simulink library "Vapour_Content"  (R2018b)
settings: Solver=ode45  StartTime=0.0  StopTime=10.0  RelTol=1e-3  EnableMultiTasking=on
undefined symbols (not defined in the file): CarnotCallbacks_Vapour_Content
settings Model: Creator=lena.frank  LastModifiedBy=P41573
settings DataIOCC: LimitDataPoints=on  SaveFormat=Array  SignalLoggingSaveFormat=ModelDataLogs
settings OptimizationCC: ExpressionDepthLimit=2147483647  LifeSpan=inf
settings DebuggingCC: UnderspecifiedInitializationDetection=Classic  MergeDetectMultiDrivingBlocksExec=none  SolverPrmCheckMsg=warning  FcnCallInpInsideContextMsg=warning  StateNameClashWarn=warning  SFUnexpectedBacktrackingDiag=warning  SFNoUnconditionalDefaultTransitionDiag=warning  SFExecutionAtInitializationDiag=none
settings HardwareCC: ProdBitPerPointer=32  ProdBitPerSizeT=32  ProdBitPerPtrDiffT=32  ProdLargestAtomicFloat=None  ProdIntDivRoundTo=Undefined  ProdEndianess=Unspecified  ProdWordSize=32  ProdHWDeviceType=32-bit Generic
settings ModelReferenceCC: PropagateSignalLabelsOutOfModel=off
settings SFSimCC: SimUseLocalCustomCode=off
settings RTWCC: RTWUseLocalCustomCode=off
settings CodeAppCC: StateflowObjectComments=on
settings GRTTargetCC: TargetLangStandard=C89/C90 (ANSI)  GeneratePreprocessorConditionals=Disable all  CombineOutputUpdateFcns=off  GRTInterface=on
settings ConfigComp: CovMetricSettings=dw  CovHtmlReporting=on  CovSaveCumulativeToWorkspaceVar=on  CovSaveSingleToWorkspaceVar=on  CovExternalEMLEnable=off

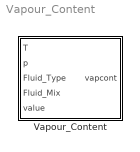
== system Vapour_Content ==
  Vapour_Content : Subsystem  LoadFcn=CarnotCallbacks_Vapour_Content('LoadFcn');  InitFcn=load('THB.mat');  VariantControl=CarlibClassic  mask(vapourcontent){INPUTARGUMENTS=state variables (classic), PROPERTYTYPE=density, DEBUGLEVEL=WARNINGLEVEL, MAXTOTALMESSAGES=inf, MAXCONSECUTIVEMESSAGES=inf, WRITETOFILE=0, FILENAME='errors.txt'}
      mask prompts: INPUTARGUMENTS "Input arguments"; PROPERTYTYPE "property type"; DEBUGLEVEL "Debug level"; MAXTOTALMESSAGES "maximum number of total warning"; MAXCONSECUTIVEMESSAGES "maximum number of consecutive warnings"; WRITETOFILE "write messages to file"; FILENAME "filename for error messages"
      mask help:
      | The block calculates the (water-)vapour content of water or water-glycol mixture by the value of a specified property. The block calls the function "vapourcontent" in the CARNOT library "Carlib".
      | Temperature and the "Value" may be a scalar or vector, all other inputs must be scalar (length of "temperature" and "value" must be same).
      | You may use the block "GlobalMessageLevel" in the Toolbox to handle the debugging messages.
      | Definition of property-types
      | property                    unit
      |  density                     [kg/m³]
      |  heat capacity           [J/kgK]
      |  heat conductivity     [W/mK]
      |  kinematic viscosity   [m²/s]
      |  enthalpy                   [J/kg]
      |  entropy                     [J/kgK]
      |  prandtl                      [-]
      |  specific volume        [m³/kg]
      mask init:
      | %Inports
      | CarnotCallbacks_Vapour_Content('CreateInports');
      | 
      | %global debug level
      | [DEBUGLEVEL, MAXTOTALMESSAGES, MAXCONSECUTIVEMESSAGES, WRITETOFILE, FILENAME] = CarnotCallbacks_Vapour_Content('CheckDebugLevels', DEBUGLEVEL, MAXTOTALMESSAGES, MAXCONSECUTIVEMESSAGES, WRITETOFILE, FILENAME);
      mask Help: web(fullfile(path_carnot('help'),'vapour_content.html'),'-helpbrowser')
      mask TypeOptions INPUTARGUMENTS: state variables (classic) | THB | THV
      mask Callback INPUTARGUMENTS: CarnotCallbacks_Vapour_Content('MaskVisibilities');
      mask TypeOptions PROPERTYTYPE: density | heat capacity | heat conductivity | kinematic viscosity | enthalpy | entropy | prandtl | specific volume
      mask TypeOptions DEBUGLEVEL: DEBUGLEVEL | INFOLEVEL | WARNINGLEVEL | ERRORLEVEL | FATALLEVEL | NOLEVEL
      mask DialogControl ParameterTabVar0 Prompt: Parameters
      mask DialogControl ParameterTabVar01 Prompt: Debugging

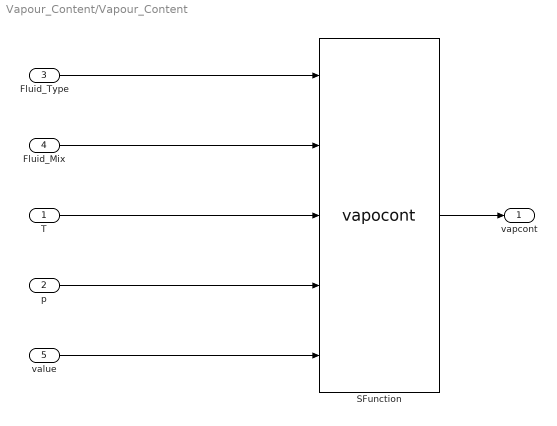
== system Vapour_Content/Vapour_Content ==
  T : Inport
  p : Inport  Port=2
  Fluid_Type : Inport  Port=3
  Fluid_Mix : Inport  Port=4
  value : Inport  Port=5
  SFunction : S-Function  FunctionName=vapocont  Parameters=PROPERTYTYPE, DEBUGLEVEL, MAXTOTALMESSAGES, MAXCONSECUTIVEMESSAGES,WRITETOFILE, FILENAME  SFunctionDeploymentMode=off  EnableBusSupport=off
  vapcont : Outport
  wires:
  SFunction/1 -> vapcont/1
  T/1 -> SFunction/3
  p/1 -> SFunction/4
  Fluid_Type/1 -> SFunction/1
  Fluid_Mix/1 -> SFunction/2
  value/1 -> SFunction/5
